simulink model "bus_creator_vs_mux"  (R2018b)
settings: Solver=VariableStepAuto  StartTime=0.0  StopTime=10.0  RelTol=1e-3
settings Model: Creator=marwan  LastModifiedBy=marwan

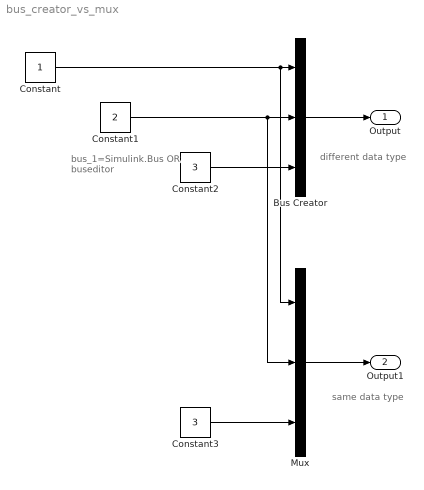
== system bus_creator_vs_mux ==
  note: same data type
  note: bus_1=Simulink.Bus
      | OR
      | buseditor
  note: different data type
  Bus Creator : BusCreator  Inputs=3  OutDataTypeStr=Bus:bus_1
  Constant : Constant  OutDataTypeStr=int16
  Constant1 : Constant  Value=2  OutDataTypeStr=int16
  Constant2 : Constant  Value=3  OutDataTypeStr=uint16
  Constant3 : Constant  Value=3  OutDataTypeStr=int16
  Mux : Mux  Inputs=3
  Output : Outport  OutDataTypeStr=Bus:bus_1
  Output1 : Outport  Port=2
  wires:
  Constant2/1 -> Bus Creator/3
  Constant1/1 -> Mux/2, Bus Creator/2
  Constant/1 -> Mux/1, Bus Creator/1
  Mux/1 -> Output1/1
  Constant3/1 -> Mux/3
  Bus Creator/1 -> Output/1
